simulink model "AR_Drone_Flight_Control"  (R2014a)
settings: configuration reference "AR_Drone_ConfigSet" (kept outside this file)
values from neighbouring files (symbols this model uses):
  Accelerometer_quick_calibration = [0.003485 0.008674 -0.9985]    [Calibration_Parameters.mat]
  Gyrometer_quick_calibration = [-10.63 2.778 -0.1868]    [Calibration_Parameters.mat]
undefined symbols (not defined in the file or in its folder): Accelerometer_360deg_calibration, Drone_StateModeType, Magnetometer_calibration, Navigation, Navigation_KF_Lib, sigbuilder_block
libraries: simulink x15, vrlib x7, aerolibtransform2 x5, AR_Drone_2_Library x4, dspnetwork x3, aerolibutil x2
(part 2 of 3)

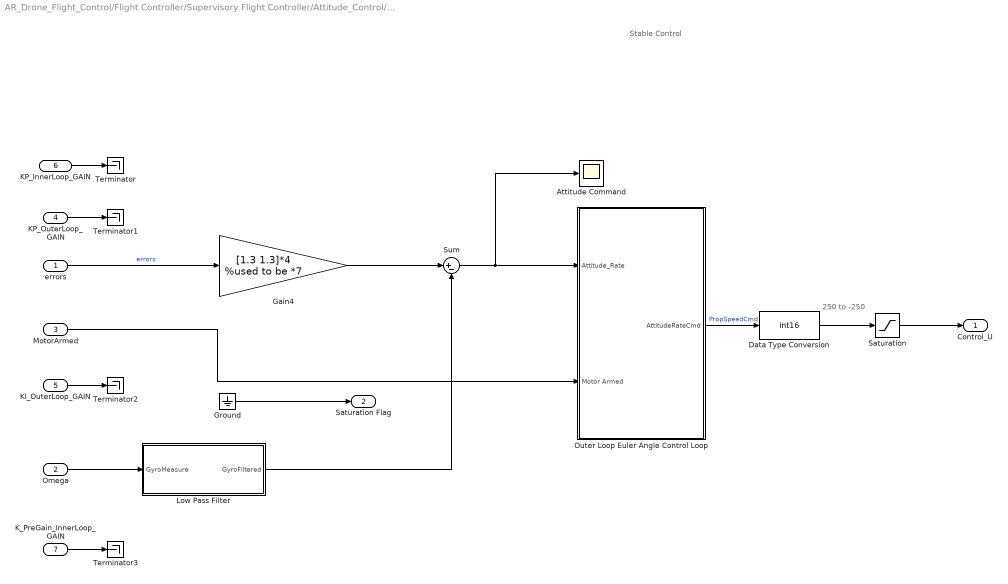
== system AR_Drone_Flight_Control/Flight Controller/Supervisory Flight Controller/Attitude_Control/Roll Pitch Controller ==
  note: 250 to -250
  note: Stable Control
  errors : Inport
  Omega : Inport  Port=2
  MotorArmed : Inport  Port=3
  KP_OuterLoop_GAIN : Inport  Port=4
  KI_OuterLoop_GAIN : Inport  Port=5
  KP_InnerLoop_GAIN : Inport  Port=6
  K_PreGain_InnerLoop_GAIN : Inport  Port=7
  Attitude Command : Scope
      settings: SaveName=AttitudeRateCtrl_Cmd
  Data Type Conversion : DataTypeConversion  OutDataTypeStr=int16  RndMeth=Nearest
  Gain4 : Gain  Gain="[1.3 1.3]*4  %used to be *7"
  Ground : Ground
  Low Pass Filter : Subsystem
  Outer Loop Euler Angle Control Loop : Subsystem
  Saturation : Saturate  UpperLimit=250  LowerLimit=-250  OutDataTypeStr=int16
      settings: AttributesFormatString=%<LowerLimit>\nto\n%<UpperLimit>
  Sum : Sum  Inputs=|+-
  Terminator{,1..3} (4 alike) : Terminator
  Control_U : Outport
  Saturation Flag : Outport  Port=2
  wires:
  Saturation/1 -> Control_U/1
  Data Type Conversion/1 -> Saturation/1
  Outer Loop Euler Angle Control Loop/1(AttitudeRateCmd) -> Data Type Conversion/1  "PropSpeedCmd"
  MotorArmed/1 -> Outer Loop Euler Angle Control Loop/2(Motor Armed)
  Ground/1 -> Saturation Flag/1
  Omega/1 -> Low Pass Filter/1(GyroMeasure)
  errors/1 -> Gain4/1  "errors"
  Sum/1 -> Attitude Command/1, Outer Loop Euler Angle Control Loop/1(Attitude_Rate)
  Gain4/1 -> Sum/1
  Low Pass Filter/1(GyroFiltered) -> Sum/2
  KP_InnerLoop_GAIN/1 -> Terminator/1
  KP_OuterLoop_GAIN/1 -> Terminator1/1
  KI_OuterLoop_GAIN/1 -> Terminator2/1
  K_PreGain_InnerLoop_GAIN/1 -> Terminator3/1

== system AR_Drone_Flight_Control/Flight Controller/Supervisory Flight Controller/Attitude_Control/Yaw Counter-Active Control ==
  note: This Yaw Controller will prevent the drone from
      | rotating but does not tell the drone to rotate to a specified angle
  Euler_Yaw_Deg : Inport
  Rate_Gyro_R_deg : Inport  Port=2
  "Desired_yaw " : Inport  Port=3
  Add1 : Sum  Inputs=+-  AccumDataTypeStr=single  OutDataTypeStr=single
  Add2 : Sum  Inputs=+-  AccumDataTypeStr=single  OutDataTypeStr=single
  Data Type Conversion : DataTypeConversion  OutDataTypeStr=int16
  Discrete Derivative : simulink/Discrete/Discrete Derivative  gainval=1.0  ICPrevScaledInput=0.0  InputProcessing=Inherited  OutMin=[]  OutMax=[]  OutDataType=fixdt(1, 16)  OutScaling=2^-10  DoSatur=off
  InterChange_Axis : Gain  Gain=-1  ParamDataTypeStr=single  OutDataTypeStr=single
      settings: AttributesFormatString=%<Gain>
  To Degrees2 : Gain  Gain=180/pi  ParamDataTypeStr=single  OutDataTypeStr=single
      settings: AttributesFormatString=%<Gain>
  To Degrees3 : Gain  ParamDataTypeStr=single  OutDataTypeStr=single
      settings: AttributesFormatString=%<Gain>
  Yaw_contribution : Gain  Gain=2.5*2  ParamDataTypeStr=single  OutDataTypeStr=single
      settings: AttributesFormatString=%<Gain>
  Yaw_contribution1 : Gain  Gain=0.06  ParamDataTypeStr=single  OutDataTypeStr=single
      settings: AttributesFormatString=%<Gain>
  YawCommand : Outport
  wires:
  Yaw_contribution1/1 -> Data Type Conversion/1
  To Degrees3/1 -> Add1/2
  Euler_Yaw_Deg/1 -> InterChange_Axis/1
  Add1/1 -> Yaw_contribution1/1
  Yaw_contribution/1 -> Add1/1
  Add2/1 -> Yaw_contribution/1
  InterChange_Axis/1 -> Discrete Derivative/1
  Discrete Derivative/1 -> Add2/1
  To Degrees2/1 -> Add2/2
  "Desired_yaw "/1 -> To Degrees2/1
  Rate_Gyro_R_deg/1 -> To Degrees3/1
  Data Type Conversion/1 -> YawCommand/1

== system AR_Drone_Flight_Control/Flight Controller/Supervisory Flight Controller/Attitude_Control/Yaw Signal Builder  ==
  Demux : Demux  Tag=STV Demux  Outputs=1
  FromWs : FromWorkspace  Tag=STV FromWs  VariableName=tuvar
      SigBuilderData=|
      | common.afterFinalStr = 'Extrapolate'
      | common.sampleTime = '-1'
      | dataSet.timeRange = [0 20]
      | dataSet.name = 'Group 1'
      | sbobj.Groups.Name = 'Group 1'
      | sbobj.Groups.Signals.Name = 'Signal 1'
      | sbobj.Groups.Signals.XData = [0 10 10 12.5 12.5 15 15 20]
      | sbobj.Groups.Signals.YData = [0 0 2 2 -2 -2 0 0]
      | sbobj.Groups.TimeRange = [0 20]
  Signal 1 : Outport  Tag=STV Outport
  wires:
  Demux/1 -> Signal 1/1
  FromWs/1 -> Demux/1

== stateflow chart AR_Drone_Flight_Control/Navigation/CheckSum Pre-Processing/Ultrasound Processing/CheckSum Correction/Generate Sample Holding Pulse/Chart ==
  state Begin_State0
    entry: output =0;
  state Begin_State
    entry: output =1;
  state End_State
    entry: output=0;
  (default) -> Begin_State0
  Begin_State0 -> Begin_State : [if_transition==1]
  Begin_State -> End_State [order 1] : after(HoldDataTicks,tick)
  End_State -> Begin_State : [if_transition==1]
  Begin_State -> Begin_State [order 2] : [if_transition==1]
  data: output output; if_transition input; HoldDataTicks input

== matlab function AR_Drone_Flight_Control/Navigation/CheckSum Pre-Processing/Ultrasound Processing/Height Calculation ==
  data: u input double; y output double; prev_good_height output double; z_1 input double
function [y,prev_good_height] = fcn(u,z_1)
%#codegen



if u<10000
    
    height = ((u - 880) /26.553);
    prev_good_height = height;
else
    
%     height = u;
%     prev_good_height = height;
    height =  z_1;
    prev_good_height = z_1; 
end

y = height;

== stateflow chart AR_Drone_Flight_Control/Flight Controller/Supervisory Flight Controller ==
  state Fault_Check [parallel]
    settings: executionOrder=3
    state BatteryFault_Check [parallel]
      settings: executionOrder=1
      state BatteryNominal
        en:
        BatteryFault = 0;
        state Nominal
        note: Description:
            | This state will be responsible for the following
            |
            | - Automatically land the drone by forcing it to the land state when voltage is low
            | - Prevent drone from taking off if battery voltage is too low
        state EvaluateVoltageLevel
        state ChangeState
          en:
          BatteryFault = 1;
        EvaluateVoltageLevel -> Fault_Check.BatteryFault_Check.BatteryNominal.Nominal [order 1] : [Measured_Battery_Voltage>=10.1]
        Fault_Check.BatteryFault_Check.BatteryNominal.Nominal -> EvaluateVoltageLevel : [Measured_Battery_Voltage<10.1]
        (default) -> EvaluateVoltageLevel
        EvaluateVoltageLevel -> Fault_Check.BatteryFault_Check.BatteryNominal.ChangeState [order 2] : after(5,sec)
      state BatteryLow
        state ForceLanding
          en:
        (default) -> ForceLanding
      (default) -> BatteryNominal
      BatteryNominal -> BatteryLow : [BatteryFault==1]
    state UltraSoundwarning_Check [parallel]
      settings: executionOrder=2
    state SafeOrientation_Check [parallel]
      settings: executionOrder=3
      state UnsafeOrientation
        du:
        MotorArmed =0;
        LandingPhase = 0;
      state WaitForFlight
      state GravityVectorCheck
        en:
        OrientationFault = 0;
        note: Description:
            | This state will be responsible for the following
            |
            | - Automatically land the drone by forcing it to the land state when voltage is low
            | - Prevent drone from taking off if battery voltage is too low
        state Nominal
        state EvaluateGravityVector
        state ChangeState
          en:
          OrientationFault = 1;
        EvaluateGravityVector -> Fault_Check.SafeOrientation_Check.GravityVectorCheck.Nominal [order 1] : [AccelVector_Input<-0.05]
        Fault_Check.SafeOrientation_Check.GravityVectorCheck.Nominal -> EvaluateGravityVector : [AccelVector_Input>=0.05]
        (default) -> EvaluateGravityVector
        EvaluateGravityVector -> Fault_Check.SafeOrientation_Check.GravityVectorCheck.ChangeState [order 2] : after(0.01,sec)
      (default) -> WaitForFlight
      GravityVectorCheck -> WaitForFlight [order 2] : [in(Drone_State.WaitForHost)]
      GravityVectorCheck -> UnsafeOrientation [order 1] : [OrientationFault ==1]
      WaitForFlight -> GravityVectorCheck : [in(Drone_State.Controlled_Flight)]
  state Drone_State [parallel]
    settings: executionOrder=1
    state WaitForHost
      entry:
      reset_offset_calc = 0;
      MotorArmed = 0;
      refHeight = 0;
      LandingPhase = 0;
      Flight_Mission_On_Off = false;
      note: Description:
          | -This state will wait for the host command to take off, while initializing the offsets (accel & gyro)
          |
          | -Upon entry, this block will set the motor to NOT ARMED (turn off integrators in controller, set safety clamp of motors to OFF)
          | -Upon entry, set the refHeight to ZERO
          | -Upon entry, reset the offset calculation such that we can re-start the averaging block
      state converge = checkConvergence(Euler_Angles) [function]
      state move = checkMove(Euler_Angles) [function]
      state Attitude_Convergence_Wait
        entry:
        initDone=false;
        during:
        Converge_Flag = checkConvergence(Gyro_Measures_for_Offset);
      state Calculate_Attitude_Offset
        entry:
        reset_offset_calc = 0 ;
        Move = false;
        during:
        Offset_Accel_Current =Accel_Offset_Calculation(Accel_Measures_for_Offset,reset_offset_calc);
        Offset_Gyro_Current =Gyro_Offset_Calculation(Gyro_Measures_for_Offset,reset_offset_calc);
        Move = checkMove(Gyro_Measures_for_Offset);
      state Wait_For_Flight
        entry:
        Offset_Accel = Accelerometer_quick_calibration;
        Offset_Gyro = Gyrometer_quick_calibration;
        during:
        initDone = true;
      state Auto_Calibration_Done
        entry:
        Offset_Accel = Offset_Accel_Current;
        Offset_Gyro = Offset_Gyro_Current;
        reset_offset_calc = 1;
        Accel_Offset_Calculation(Accel_Measures_for_Offset,reset_offset_calc);
        Gyro_Offset_Calculation(Gyro_Measures_for_Offset,reset_offset_calc);
        during:
        initDone = true;
      (default) -> Attitude_Convergence_Wait
      Calculate_Attitude_Offset -> Attitude_Convergence_Wait [order 2] : [Move == 1 && after(0.1,sec)]
          | {reset_offset_calc = 1;
          | Accel_Offset_Calculation(Accel_Measures_for_Offset,reset_offset_calc);
          | Gyro_Offset_Calculation(Gyro_Measures_for_Offset,reset_offset_calc)}
      Auto_Calibration_Done -> Attitude_Convergence_Wait [order 2] : [Auto_Calibration==false]
      Wait_For_Flight -> Attitude_Convergence_Wait : [Auto_Calibration==true]
      Attitude_Convergence_Wait -> (junction 628) : [Converge_Flag==1 && after(0.1,sec)]
      (junction 628) -> Calculate_Attitude_Offset [order 1] : [Auto_Calibration==true]
      (junction 628) -> Wait_For_Flight [order 2] : [Auto_Calibration==false]
      Calculate_Attitude_Offset -> Auto_Calibration_Done [order 1] : [Move == 0 && after(3,sec)]
      Auto_Calibration_Done -> Calculate_Attitude_Offset [order 1] : [initDone == 1 && after(0.1,sec)]
    state Controlled_Flight
      entry:
      LandingPhase = 0;
      MotorArmed =1;
      note: Description:
          | -Upon entry, this block will set the motor to ARMED (enable controller integrator and motor safetey unclamped)
          | -This block will command the AR Drone to fly up to a certain height using the variable refHeight
          | -The output of refHeight should be a function of desired Altitude. The most primitive assignment is to make refHeight = DesiredAltitude, this is comparable to giving the drone a step response. Alternate methods could be giving it a smooth trajectory to follow from the ground to that particular height
          |
          | -Below is an example of what it might look like
      state Initialize
        entry: refHeight = 0;
      state Altitude_Climb
        entry: Flight_Mission_On_Off = true;
        during: Input_ports = [0 ; 0];
        refHeight = Output_ports(2);
      (default) -> Initialize
      Initialize -> Altitude_Climb : [after(0.5,sec)]
    state Landing_Sequence
      entry:
      refHeight = min(refHeight,40);
      Flight_Mission_On_Off = false;
      note: Description:
          | -Entry into this state will occur if
          | a) Battery drops to around 10.5-10.2 Volts (needs to be experimentally validated)
          | b) Entry condition is met from the user input
          | c) Attitude is out of bounds, ie: the quad rotor has tilted it's pitch to some uncontrollable angle such as 80 degrees
          |
          | Substate goals:
          | -Descend at a controllable rate and land safely
      state Climb_down_1
        entry: refHeight = refHeight - 2 ;
      state Climb_down_2
        entry: refHeight = refHeight - 1 ;
      state Climb_down_3
        entry: LandingPhase=1;
      (default) -> Climb_down_1
      Climb_down_1 -> Climb_down_1 [order 1] : [UltraSound_Feedback(1) <= refHeight && after(0.05,sec)]
      Climb_down_1 -> Climb_down_2 [order 2] : [UltraSound_Feedback(1) <= 10 && after(0.1,sec)]
      Climb_down_2 -> Climb_down_2 [order 1] : [UltraSound_Feedback(1) <= refHeight && after(0.1,sec)]
      Climb_down_2 -> Climb_down_3 [order 2] : [UltraSound_Feedback(1) <= 0.5 && after(0.1,sec)]
    state Landing_Terminate
      entry:
      MotorArmed =0;
      LandingPhase = 0;
      Flight_Mission_On_Off = false;
      %Catch any last state action we need to do here
      note: Description:
          | This state is optional and might not be needed. Up to you if you think having an extra state for the landing phase might be useful.. if not, delete it and consolidate it into previous state
    (default) -> WaitForHost
    Landing_Terminate -> WaitForHost : [sum(MotorCmd)==0]
    WaitForHost -> Controlled_Flight : [ (hostCmd == Drone_StateModeType.Controlled_Flight)...
        |  &&...
        |  in(Fault_Check.BatteryFault_Check.BatteryNominal.Nominal)...
        | && (initDone == 1) ]
    Controlled_Flight -> Landing_Terminate [order 2] : [in(Fault_Check.SafeOrientation_Check.UnsafeOrientation)]
    Controlled_Flight -> Landing_Sequence [order 1] : [(hostCmd == ...
        | Drone_StateModeType.Landing_Sequence)...
        | ||...
        |  in(Fault_Check.BatteryFault_Check.BatteryLow) ]
    Landing_Sequence -> Landing_Terminate : [sum(MotorCmd)==0]
  state Flight_Controls [parallel]
    settings: executionOrder=2
    state Attitude_Command [parallel]
      entry, during:
      Attitude_Thrust = Attitude_Control(Desired_Attitude_deg,Euler_Angles,Angular_Velocity,MotorArmed);
      settings: executionOrder=1
    state Altitude_Command [parallel]
      entry, during:
      Altitude_Thrust = Altitude_Control(UltraSound_Feedback,refHeight);
      settings: executionOrder=2
    state MotorMixing_Command [parallel]
      entry, during:
      throttle = NominalThrust+EnableAltitudeCtrl*Altitude_Thrust;
      MotorCmd = Motor_Mixing(throttle,Attitude_Thrust,LandingPhase,MotorArmed);
      settings: executionOrder=3
  state deltaThrottle = Altitude_Control(HeightFeedback,refHeight) [function]
  state controls = Attitude_Control(Desired_Attitude_Deg,EulerAngle_Feedback_Deg,RateGyro_Feedback_Deg,Motor_Armed) [function]
  state MotorCommands = Motor_Mixing(throttle,RPYCmd,LandingPhase,Motor_Armed) [function]
  data: Euler_Angles function_input double size=3; converge function_output; OffsetMeasure function_input; Reset function_input; Y function_output; OffsetMeasure function_input; Reset function_input; Y function_output; Euler_Angles function_input double size=3; move function_output; HeightFeedback function_input double size=2; refHeight function_input double size=1; deltaThrottle function_output int16; Desired_Attitude_Deg function_input double size=3; EulerAngle_Feedback_Deg function_input double size=3; RateGyro_Feedback_Deg function_input double size=3; Motor_Armed function_input double size=1; controls function_output int16 size=3; throttle function_input int16 size=1; RPYCmd function_input int16 size=3; LandingPhase function_input double size=1; MotorCommands function_output; Motor_Armed function_input double size=1; hostCmd input Enum: Drone_StateModeType; Auto_Calibration input; EnableAltitudeCtrl input; Desired_Attitude_deg input size=3; UltraSound_Feedback input size=2; initDone local; MotorCmd output size=4; throttle local int16; deltaThrottle local; height local; Euler_Angles input; Angular_Velocity input; AccelVector_Input input; hoverHeight local; NominalThrust input; Drone_StateMode output Enum: Drone_StateModeType; Measured_Battery_Voltage input; Attitude_Thrust local; Altitude_Thrust local; Converge_Flag local; reset_offset_calc local; MotorArmed local; Offset_Accel data_store_memory; LandingPhase local; N local; Accel_Measures_for_Offset input size=3; Gyro_Measures_for_Offset input size=3; Offset_Gyro data_store_memory; Offset_Gyro_Current local; Offset_Value_Current local; Offset_Accel_Current local double; BatteryFault local; OrientationFault local; BatteryFault_Mode output Enum: BatteryFault_ModeType; SafeOrientation_Mode output Enum: SafeOrientation_ModeType; refHeight output; Move local; Landing_Altitude local; Actual_Attitude local; Gyrometer_quick_calibration parameter; Accelerometer_quick_calibration parameter; Flight_Mission_On_Off data_store_memory; Output_ports data_store_memory; Input_ports data_store_memory
  data hostCmd settings: description=|
      | The hostCmd can take the values 0,1 and 2.
      | 
      | 0 - default state when the drone is powered up.
      | 1 - Takeoff
      | 2 - Landing
  data EnableAltitudeCtrl settings: description=A flag to enable the altitude controller
  data UltraSound_Feedback settings: description=Ultrasound Feedback will contain data on current height (cm) and altitude rate (cm/s)
  data initDone settings: description=A flag to check whether the calibration is done.
  data NominalThrust settings: description=Nominal thrust input (approximately 60% duty cycle)
  data refHeight settings: description=Desired height at which the drone needs to hover.
  function Y = Accel_Offset_Calculation(OffsetMeasure,Reset):
    | function Y = Accel_Offset_Calculation(OffsetMeasure,Reset)
    |  
    | %Compute running average while in this state. Assumed inputs
    | %are accelerometer offset values. These values are accumulated over time
    | %and divided by the total time increment to return an average values
    | Y = [0 0 0]';
    | persistent A_x_sum
    | persistent A_y_sum
    | persistent A_z_sum
    | persistent Tick
    | 
    | if(isempty(A_x_sum) || Reset==1)
    |     A_x_sum = 0;
    |     A_y_sum = 0;
    |     A_z_sum = 0;
    |     Tick = 1;
    |         
    | else
    |     
    |     Measure_X = OffsetMeasure(1);
    |     Measure_Y = OffsetMeasure(2);
    |     Measure_Z = OffsetMeasure(3);
    | 
    |     A_x_sum = A_x_sum + Measure_X;
    |     A_y_sum = A_y_sum + Measure_Y;
    |     A_z_sum = A_z_sum + Measure_Z;
    | 
    | 
    |     Y = [A_x_sum A_y_sum A_z_sum]'./Tick;
    | 
    | 
    |     Tick = Tick + 1;
    | 
    | end
    | 
    | 
    | 
    | 
    | end
  function Y = Gyro_Offset_Calculation(OffsetMeasure,Reset):
    | function Y = Gyro_Offset_Calculation(OffsetMeasure,Reset)
    |  
    | %Compute running average while in this state. Assumed inputs
    | %are gyro offset values when drone is perfectly stationary on the ground. These values are accumulated over time
    | %and divided by the total time increment to return an average values
    | Y = [0 0 0]';
    | persistent G_x_sum
    | persistent G_y_sum
    | persistent G_z_sum
    | persistent Tick
    | 
    | if(isempty(G_x_sum) || Reset==1)
    |     G_x_sum = 0;
    |     G_y_sum = 0;
    |     G_z_sum = 0;
    | 
    |     Tick = 1;
    |         
    | else
    |     
    |     Measure_X = OffsetMeasure(1);
    |     Measure_Y = OffsetMeasure(2);
    |     Measure_Z = OffsetMeasure(3);
    | 
    |     G_x_sum = G_x_sum + Measure_X;
    |     G_y_sum = G_y_sum + Measure_Y;
    |     G_z_sum = G_z_sum + Measure_Z;
    | 
    | 
    |     Y = [G_x_sum G_y_sum G_z_sum]'./Tick;
    | 
    | 
    |     Tick = Tick + 1;
    | 
    | end
    | 
    | 
    | 
    | 
    | end

== system AR_Drone_Flight_Control/Flight Mission/Desired Drone_StateMode Management/Data Correction ==
  note: This Subsystem tests if the data is normal (it should be equal to -1 or +1)
      | If not (for exemple if the UDP server waits data but receives nothing : 0),
      | it affects to the data the last "normal" value seen (initial condition : -1)
  Start/Stop : Inport
  Constant1 : Constant  Value=-1
  Constant2 : Constant  Value=+1
  Logical Operator : Logic  Operator=OR  AllPortsSameDT=off  OutDataTypeStr=boolean
  Memory : Memory  X0=-1
  Switch1 : Switch  Criteria=u2 > Threshold
  Tests if data equals +1 : RelationalOperator  Operator===  OutDataTypeStr=boolean
  Tests if data equals -1 : RelationalOperator  Operator===  OutDataTypeStr=boolean
  Real Start/Stop : Outport
  wires:
  Start/Stop/1 -> Switch1/1, Tests if data equals -1/2, Tests if data equals +1/1
  Constant1/1 -> Tests if data equals -1/1
  Constant2/1 -> Tests if data equals +1/2
  Tests if data equals -1/1 -> Logical Operator/1
  Tests if data equals +1/1 -> Logical Operator/2
  Logical Operator/1 -> Switch1/2
  Switch1/1 -> Memory/1, Real Start/Stop/1
  Memory/1 -> Switch1/3

== system AR_Drone_Flight_Control/Navigation/CheckSum Pre-Processing/Accelerometer Processing ==
  Raw Data : Inport
  CheckSum Flag : Inport  Port=2
  Holding Value : Inport  Port=3
  Calculate Accel Data : Subsystem  Commented=through
  CheckSum Correction : Subsystem
  Processed Data : Outport
  wires:
  Holding Value/1 -> CheckSum Correction/3(Holding Value)
  Calculate Accel Data/1(Processed Accel Data) -> CheckSum Correction/1(CalculatedData)
  CheckSum Correction/1(Pre-Processed Height) -> Processed Data/1
  Raw Data/1 -> Calculate Accel Data/1(Raw Accel Data)
  CheckSum Flag/1 -> CheckSum Correction/2(CheckSumFlag)

== system AR_Drone_Flight_Control/Navigation/CheckSum Pre-Processing/Magnetometer ==
  Magnetometer : Inport
  CheckSum Flag : Inport  Port=2
  Holding Value : Inport  Port=3
  CheckSum Correction : Subsystem
  Process Raw Mag Data : Subsystem  Commented=through
  Processed Data : Outport
  wires:
  Holding Value/1 -> CheckSum Correction/3(Holding Value)
  Process Raw Mag Data/1(ProcessedData) -> CheckSum Correction/1(CalculatedData)
  Magnetometer/1 -> Process Raw Mag Data/1(Magnetometer)
  CheckSum Correction/1(Pre-Processed Data) -> Processed Data/1
  CheckSum Flag/1 -> CheckSum Correction/2(CheckSumFlag)

== system AR_Drone_Flight_Control/Navigation/CheckSum Pre-Processing/RateGyro Processing ==
  Raw Data : Inport
  CheckSum Flag : Inport  Port=2
  Holding Value : Inport  Port=3
  CheckSum Correction : Subsystem
  Process Data : Subsystem  Commented=through
  Processed Data : Outport
  wires:
  Holding Value/1 -> CheckSum Correction/3(Holding Value)
  Process Data/1(Processed Data) -> CheckSum Correction/1(CalculatedData)
  Raw Data/1 -> Process Data/1(Raw Data)
  CheckSum Correction/1(Pre-Processed Height) -> Processed Data/1
  CheckSum Flag/1 -> CheckSum Correction/2(CheckSumFlag)

== system AR_Drone_Flight_Control/Navigation/CheckSum Pre-Processing/TempFilter ==
  Magnetometer : Inport
  CheckSum Flag : Inport  Port=2
  HoldingValue : Inport  Port=3
  CheckSum Correction : Subsystem
  Process Raw Mag Data : Subsystem  Commented=through
  Processed Data : Outport
  wires:
  HoldingValue/1 -> CheckSum Correction/3(Holding Value)
  Process Raw Mag Data/1(ProcessedData) -> CheckSum Correction/1(CalculatedData)
  Magnetometer/1 -> Process Raw Mag Data/1(Magnetometer)
  CheckSum Correction/1(Pre-Processed Data) -> Processed Data/1
  CheckSum Flag/1 -> CheckSum Correction/2(CheckSumFlag)

== system AR_Drone_Flight_Control/Navigation/CheckSum Pre-Processing/Ultrasound Processing ==
  note: '192.168.1.1' 1 17725
  Raw Ultrasound : Inport
  CheckSum Flag : Inport  Port=2
  Holding Value : Inport  Port=3
  CheckSum Correction : Subsystem
  Data Type Conversion1 : DataTypeConversion
  Delay1 : Delay  DelayLength=1  InitialCondition=0
  Height Calculation : MATLAB Function  TreatAsAtomicUnit=on
  Saturation1 : Saturate  UpperLimit=100e3  LowerLimit=0
  Processed Data : Outport
  wires:
  Holding Value/1 -> CheckSum Correction/3(Holding Value)
  Saturation1/1 -> Processed Data/1
  CheckSum Correction/1(Pre-Processed Height) -> Saturation1/1
  CheckSum Flag/1 -> CheckSum Correction/2(CheckSumFlag)
  Height Calculation/1(y) -> CheckSum Correction/1(CalculatedData)
  Raw Ultrasound/1 -> Data Type Conversion1/1
  Height Calculation/2(prev_good_height) -> Delay1/1
  Data Type Conversion1/1 -> Height Calculation/1(u)
  Delay1/1 -> Height Calculation/2(z_1)

== system AR_Drone_Flight_Control/Navigation/Data Conversion and Measurement Calculation/Calculate Gravity Vector ==
  Accel : Inport
  Accel_Offset : Inport  Port=2
  Accelerometer Neutral Gain and Offset : Subsystem
  Calibration_GainOffset : Subsystem
  Compare Calibration : Scope  NumInputPorts=2
      settings: TimeRange=6.848856838354834  YMin=-1.05~-1.05  YMax=0.05~0.1  SaveName=AccelProcessed_Record1
  Compare Filter : Scope  NumInputPorts=2
      settings: TimeRange=6.848856838354834  YMin=-0.05~-0.05  YMax=1.05~1.05  SaveName=AccelProcessed_Record2
  Compare Offset : Scope  NumInputPorts=2
      settings: TimeRange=6.848856838354834  YMin=-0.05~-1  YMax=1.05~0.05  SaveName=AccelProcessed_Record
  InitialCondition_Offset : Subsystem
  Low Pass Filter : Subsystem
  Normalize Vector : vrlib/Utilities/Normalize Vector  maxzero=0
  Accel_Norm : Outport
  wires:
  Accel_Offset/1 -> InitialCondition_Offset/2(Accel_Offset)
  Accelerometer Neutral Gain and Offset/1(Processed Accel Data) -> Compare Calibration/2, Calibration_GainOffset/1(Pre)
  Calibration_GainOffset/1(Post) -> Compare Offset/2, Compare Calibration/1, InitialCondition_Offset/1(Pre)
  Low Pass Filter/1(Filtered Accel) -> Normalize Vector/1, Compare Filter/1
  InitialCondition_Offset/1(Post) -> Low Pass Filter/1(Offset Accel), Compare Filter/2, Compare Offset/1
  Accel/1 -> Accelerometer Neutral Gain and Offset/1(Raw Accel Data)
  Normalize Vector/1 -> Accel_Norm/1

== system AR_Drone_Flight_Control/Navigation/Data Conversion and Measurement Calculation/Calibration_Scale_and_Offset ==
  RawMag : Inport
  Normalize Vector : vrlib/Utilities/Normalize Vector  maxzero=0
  Process Raw Mag Data : Subsystem  Variant=on  OverrideUsingVariant=TempVariantA
  Normalized  Magnetometer : Outport
  wires:
  Process Raw Mag Data/1(MagVector) -> Normalize Vector/1
  RawMag/1 -> Process Raw Mag Data/1(Magnetometer)
  Normalize Vector/1 -> Normalized  Magnetometer/1

== system AR_Drone_Flight_Control/Navigation/Data Conversion and Measurement Calculation/Remove Offset ==
  Raw Gyro Values : Inport
  Gyro Offset : Inport  Port=2
  BeforeAfter : Scope
      settings: YMin=-40  YMax=40
  Demux : Demux  Outputs=3
  Demux1 : Demux  Outputs=3
  Display : Display
  Mux : Mux  Inputs=2
  Mux1 : Mux  Inputs=3
  Process Raw Rate Gyro Data : Subsystem
  Sum : Sum  Inputs=|+-
  Sum1 : Sum  Inputs=|+-
  Sum2 : Sum  Inputs=|+-
  Gyro Offset Remove : Outport
  tag scope: Gyro_data_for_offset=global
  wires:
  Process Raw Rate Gyro Data/1(Processed Data) -> Gyro Offset Remove/1
  Mux/1 -> BeforeAfter/1
  Raw Gyro Values/1 -> Demux/1, Mux/1, [Gyro_data_for_offset]
  Gyro Offset/1 -> Demux1/1
  Mux1/1 -> Process Raw Rate Gyro Data/1(Raw Rate Gyro Data), Display/1, Mux/2
  Demux1/3 -> Sum2/2
  Demux1/2 -> Sum1/2
  Demux1/1 -> Sum/2
  Demux/2 -> Sum1/1
  Demux/1 -> Sum/1
  Sum1/1 -> Mux1/2
  Demux/3 -> Sum2/1
  Sum2/1 -> Mux1/3
  Sum/1 -> Mux1/1

== system AR_Drone_Flight_Control/Navigation/SL3D Visualization/Interchange Axes Accel for SL3D  ==
  VRML_in : Inport
  Demux1 : Demux  Outputs=3
  Gain1 : Gain  Gain=3
  Gain2 : Gain
  Gain3 : Gain
  Mux2 : Mux  Inputs=3
  VRML_out : Outport
  wires:
  VRML_in/1 -> Gain1/1
  Demux1/2 -> Gain2/1
  Mux2/1 -> VRML_out/1
  Gain3/1 -> Mux2/3
  Gain2/1 -> Mux2/1
  Demux1/3 -> Mux2/2
  Demux1/1 -> Gain3/1
  Gain1/1 -> Demux1/1

== system AR_Drone_Flight_Control/Navigation/SL3D Visualization/Interchange Axes Mag for SL3D  ==
  VRML_in : Inport
  Home Drone : Subsystem
  Subsystem : Subsystem  Commented=on
  Work Drone : Subsystem
  Work Drone - supposed work drone .. not really : Subsystem
  VRML_out : Outport
  wires:
  Work Drone/1(Out1) -> VRML_out/1
  VRML_in/1 -> Home Drone/1(In1), Work Drone/1(In1)

== system AR_Drone_Flight_Control/Navigation/SL3D Visualization/Interchange Axis Mag Project for SL3D ==
  VRML_in : Inport
  Demux1 : Demux  Outputs=3
  Gain2 : Gain
  Gain3 : Gain
  Mux2 : Mux  Inputs=3
  VRML_out : Outport
  wires:
  Demux1/2 -> Gain2/1
  Mux2/1 -> VRML_out/1
  Gain3/1 -> Mux2/3
  Gain2/1 -> Mux2/1
  Demux1/3 -> Mux2/2
  Demux1/1 -> Gain3/1
  VRML_in/1 -> Demux1/1

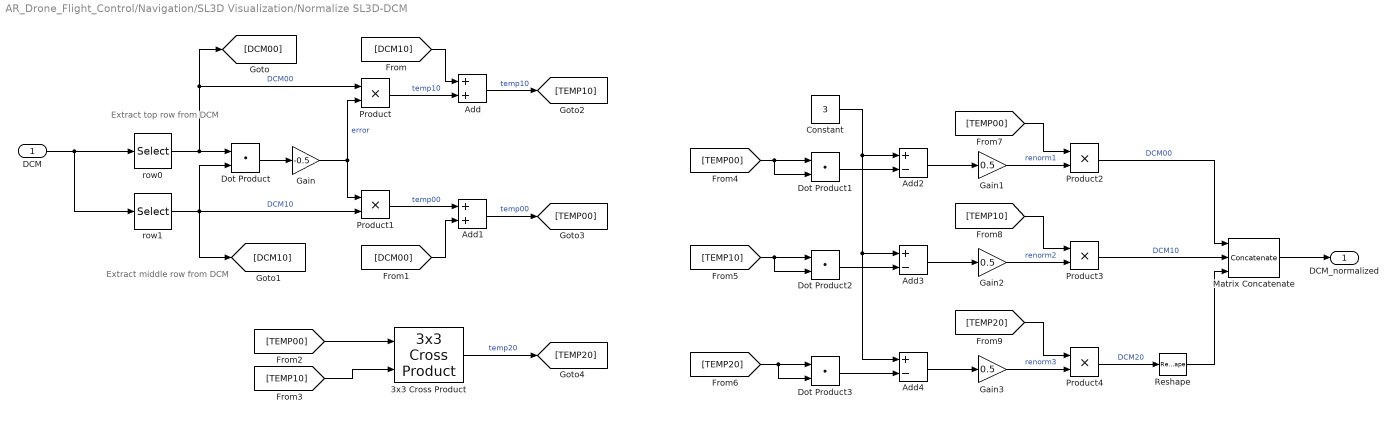
== system AR_Drone_Flight_Control/Navigation/SL3D Visualization/Normalize SL3D-DCM ==
  note: Extract top row from DCM
  note: Extract middle row from DCM
  DCM : Inport  OutDataTypeStr=double  PortDimensions=[3,3]
  3x3 Cross Product : aerolibutil/3x3 Cross Product
  Add : Sum
  Add1 : Sum
  Add2 : Sum  Inputs=+-
  Add3 : Sum  Inputs=+-
  Add4 : Sum  Inputs=+-
  Constant : Constant  Value=3  OutDataTypeStr=double  SampleTime=-1
  Dot Product{,1..3} (4 alike) : DotProduct  InputSameDT=on  OutDataTypeStr=Inherit: Inherit via internal rule
  Gain : Gain  Gain=-0.5
  Gain1 : Gain  Gain=0.5  OutDataTypeStr=single
  Gain2 : Gain  Gain=0.5  OutDataTypeStr=single
  Gain3 : Gain  Gain=0.5  OutDataTypeStr=single
  Matrix Concatenate : Concatenate  NumInputs=3  Mode=Multidimensional array
  Product{,1..4} (5 alike) : Product  RndMeth=Zero
  Reshape : Reshape  OutputDimensionality=Row vector (2-D)
  row0 : Selector  NumberOfDimensions=2  IndexMode=Zero-based  InputPortWidth=3  IndexOptions=Index vector (dialog),Index vector (dialog)  Indices=0,[0:2]  OutputSizes=1,1
  row1 : Selector  NumberOfDimensions=2  IndexMode=Zero-based  InputPortWidth=3  IndexOptions=Index vector (dialog),Index vector (dialog)  Indices=1,[0:2]  OutputSizes=1,1
  DCM_normalized : Outport  OutDataTypeStr=double
  wires:
  DCM/1 -> row0/1, row1/1
  row0/1 -> Dot Product/1, Product/1, [DCM00]  "DCM00"
  row1/1 -> Dot Product/2, Product1/2, [DCM10]  "DCM10"
  Dot Product/1 -> Gain/1
  Gain/1 -> Product/2, Product1/1  "error"
  Product/1 -> Add/2  "temp10"
  Product1/1 -> Add1/1  "temp00"
  [DCM10] -> Add/1
  [DCM00] -> Add1/2
  Add/1 -> [TEMP10]  "temp10"
  Add1/1 -> [TEMP00]  "temp00"
  3x3 Cross Product/1 -> [TEMP20]  "temp20"
  [TEMP00] -> 3x3 Cross Product/1
  [TEMP10] -> 3x3 Cross Product/2
  [TEMP00] -> Dot Product1/1, Dot Product1/2
  [TEMP10] -> Dot Product2/1, Dot Product2/2
  [TEMP20] -> Dot Product3/1, Dot Product3/2
  Dot Product1/1 -> Add2/2
  Constant/1 -> Add2/1, Add4/1, Add3/1
  Add2/1 -> Gain1/1
  Gain1/1 -> Product2/2  "renorm1"
  Add3/1 -> Gain2/1
  Gain2/1 -> Product3/2  "renorm2"
  Dot Product2/1 -> Add3/2
  Add4/1 -> Gain3/1
  Gain3/1 -> Product4/2  "renorm3"
  Dot Product3/1 -> Add4/2
  [TEMP00] -> Product2/1
  [TEMP10] -> Product3/1
  [TEMP20] -> Product4/1
  Product2/1 -> Matrix Concatenate/1  "DCM00"
  Product3/1 -> Matrix Concatenate/2  "DCM10"
  Product4/1 -> Reshape/1  "DCM20"
  Matrix Concatenate/1 -> DCM_normalized/1
  Reshape/1 -> Matrix Concatenate/3

== system AR_Drone_Flight_Control/Navigation/SL3D Visualization/SL3D DCM Output - used to adjust axes to fit wit SL3D convention ==

== system AR_Drone_Flight_Control/Data decomposition to 3D Visualization/SL3D Visualization1/Interchange Axes Mag for SL3D /Home Drone ==
  note: This comes close, however, it doesnt seem that the axis changes properly
      | ie: i rotate drone, the green dot follows it. This  tells me the Z-axis is not
      |  properly placed
  note: y
  note: x
  note: z
  In1 : Inport
  Demux1 : Demux  Outputs=3
  Gain : Gain  Gain=-1
  Gain1 : Gain
  Gain2 : Gain
  Mux2 : Mux  Inputs=3
  Out1 : Outport
  wires:
  Mux2/1 -> Out1/1
  In1/1 -> Demux1/1
  Demux1/3 -> Gain2/1
  Gain2/1 -> Mux2/2
  Demux1/1 -> Gain/1
  Gain/1 -> Mux2/3
  Demux1/2 -> Gain1/1
  Gain1/1 -> Mux2/1

== system AR_Drone_Flight_Control/Data decomposition to 3D Visualization/SL3D Visualization1/Interchange Axes Mag for SL3D /Subsystem ==
  note: This comes close, however, it doesnt seem that the axis changes properly
      | ie: i rotate drone, the green dot follows it. This  tells me the Z-axis is not
      |  properly placed
  note: y
  note: x
  note: z
  In1 : Inport
  Demux1 : Demux  Outputs=3
  Gain : Gain
  Gain1 : Gain  Gain=-1
  Gain2 : Gain  Gain=-1
  Mux2 : Mux  Inputs=3
  Out1 : Outport
  wires:
  Demux1/1 -> Gain2/1
  Gain2/1 -> Mux2/2
  Gain/1 -> Mux2/3
  Gain1/1 -> Mux2/1
  Mux2/1 -> Out1/1
  Demux1/2 -> Gain1/1
  Demux1/3 -> Gain/1
  In1/1 -> Demux1/1

== system AR_Drone_Flight_Control/Data decomposition to 3D Visualization/SL3D Visualization1/Interchange Axes Mag for SL3D /Work Drone ==
  note: This comes close, however, it doesnt seem that the axis changes properly
      | ie: i rotate drone, the green dot follows it. This  tells me the Z-axis is not
      |  properly placed
  note: y
  note: x
  note: z
  In1 : Inport
  Demux1 : Demux  Outputs=3
  Gain : Gain  Gain=-1
  Gain1 : Gain
  Gain2 : Gain
  Mux2 : Mux  Inputs=3
  Out1 : Outport
  wires:
  Mux2/1 -> Out1/1
  In1/1 -> Demux1/1
  Demux1/3 -> Gain2/1
  Gain2/1 -> Mux2/2
  Demux1/1 -> Gain/1
  Gain/1 -> Mux2/3
  Demux1/2 -> Gain1/1
  Gain1/1 -> Mux2/1

== system AR_Drone_Flight_Control/Data decomposition to 3D Visualization/SL3D Visualization1/Interchange Axes Mag for SL3D /Work Drone - supposed work drone .. not really ==
  note: This comes close, however, it doesnt seem that the axis changes properly
      | ie: i rotate drone, the green dot follows it. This  tells me the Z-axis is not
      |  properly placed
  note: y
  note: x
  note: z
  In1 : Inport
  Demux1 : Demux  Outputs=3
  Gain : Gain  Gain=-1
  Gain1 : Gain
  Gain2 : Gain  Gain=-1
  Mux2 : Mux  Inputs=3
  Out1 : Outport
  wires:
  Mux2/1 -> Out1/1
  In1/1 -> Demux1/1
  Demux1/3 -> Gain2/1
  Gain2/1 -> Mux2/2
  Demux1/1 -> Gain/1
  Gain/1 -> Mux2/3
  Demux1/2 -> Gain1/1
  Gain1/1 -> Mux2/1

== system AR_Drone_Flight_Control/Flight Controller/Supervisory Flight Controller/Attitude_Control/Roll Pitch Controller/Low Pass Filter ==
  GyroMeasure : Inport
  Demux : Demux  Outputs=2
  Digital Low Pass Filter1 : DiscreteTransferFcn  Numerator=[0.04877]  Denominator=[1 -0.9512]  OutDataTypeStr=int16
  Digital Low Pass Filter2 : DiscreteTransferFcn  Numerator=[0.04877]  Denominator=[1 -0.9512]  OutDataTypeStr=int16
  Digital Low Pass Filter3 : DiscreteTransferFcn  Commented=on  Numerator=[0.04877]  Denominator=[1 -0.9512]  OutDataTypeStr=int16
  Mux3 : Mux  Inputs=2
  GyroFiltered : Outport
  wires:
  Mux3/1 -> GyroFiltered/1
  Demux/1 -> Digital Low Pass Filter2/1
  GyroMeasure/1 -> Demux/1
  Demux/2 -> Digital Low Pass Filter1/1
  Digital Low Pass Filter2/1 -> Mux3/1
  Digital Low Pass Filter1/1 -> Mux3/2

== system AR_Drone_Flight_Control/Flight Controller/Supervisory Flight Controller/Attitude_Control/Roll Pitch Controller/Outer Loop Euler Angle Control Loop ==
  Attitude_Rate : Inport
  Motor Armed : Inport  Port=2
  Logical Operator : Logic  Operator=NOT  AllPortsSameDT=off  OutDataTypeStr=boolean
  PID Controller : simulink/Continuous/PID Controller  Controller=PID  TimeDomain=Discrete-time  SampleTime=-1  IntegratorMethod=Forward Euler  FilterMethod=Forward Euler  Form=Parallel  P=2.8281  I=28.23  D=0.023379  N=0.0076593  InitialConditionSource=internal  InitialConditionForIntegrator=0  InitialConditionForFilter=0  ExternalReset=level  LimitOutput=on  UpperSaturationLimit=30  LowerSaturationLimit=-30  LinearizeAsGain=on  AntiWindupMode=clamping  Kb=1  TrackingMode=off  Kt=1  PParamMin=[]  PParamMax=[]  IParamMin=[]  IParamMax=[]  DParamMin=[]  DParamMax=[]  NParamMin=[]  NParamMax=[]  KbParamMin=[]  KbParamMax=[]  KtParamMin=[]  KtParamMax=[]  POutMin=[]  POutMax=[]  IOutMin=[]  IOutMax=[]  DOutMin=[]  DOutMax=[]  NOutMin=[]  NOutMax=[]  KbOutMin=[]  KbOutMax=[]  KtOutMin=[]  KtOutMax=[]  IntegratorOutMin=[]  IntegratorOutMax=[]  FilterOutMin=[]  FilterOutMax=[]  SumOutMin=[]  SumOutMax=[]  SumI1OutMin=[]  SumI1OutMax=[]  SumI2OutMin=[]  SumI2OutMax=[]  SumI3OutMin=[]  SumI3OutMax=[]  SumDOutMin=[]  SumDOutMax=[]  SaturationOutMin=[]  SaturationOutMax=[]  IntegratorContinuousStateAttributes=''  IntegratorStateMustResolveToSignalObject=off  IntegratorRTWStateStorageClass=Auto  FilterContinuousStateAttributes=''  FilterStateMustResolveToSignalObject=off  FilterRTWStateStorageClass=Auto
  PID Controller1 : simulink/Continuous/PID Controller  Controller=PID  TimeDomain=Discrete-time  SampleTime=-1  IntegratorMethod=Forward Euler  FilterMethod=Forward Euler  Form=Parallel  P=0.10084*2  I=0.13631*2  D=-0.011755  N=5  InitialConditionSource=internal  InitialConditionForIntegrator=0  InitialConditionForFilter=0  ExternalReset=level  LimitOutput=on  UpperSaturationLimit=30  LowerSaturationLimit=-30  LinearizeAsGain=on  AntiWindupMode=clamping  Kb=1  TrackingMode=off  Kt=1  PParamMin=[]  PParamMax=[]  IParamMin=[]  IParamMax=[]  DParamMin=[]  DParamMax=[]  NParamMin=[]  NParamMax=[]  KbParamMin=[]  KbParamMax=[]  KtParamMin=[]  KtParamMax=[]  POutMin=[]  POutMax=[]  IOutMin=[]  IOutMax=[]  DOutMin=[]  DOutMax=[]  NOutMin=[]  NOutMax=[]  KbOutMin=[]  KbOutMax=[]  KtOutMin=[]  KtOutMax=[]  IntegratorOutMin=[]  IntegratorOutMax=[]  FilterOutMin=[]  FilterOutMax=[]  SumOutMin=[]  SumOutMax=[]  SumI1OutMin=[]  SumI1OutMax=[]  SumI2OutMin=[]  SumI2OutMax=[]  SumI3OutMin=[]  SumI3OutMax=[]  SumDOutMin=[]  SumDOutMax=[]  SaturationOutMin=[]  SaturationOutMax=[]  IntegratorContinuousStateAttributes=''  IntegratorStateMustResolveToSignalObject=off  IntegratorRTWStateStorageClass=Auto  FilterContinuousStateAttributes=''  FilterStateMustResolveToSignalObject=off  FilterRTWStateStorageClass=Auto
  AttitudeRateCmd : Outport
  wires:
  PID Controller1/1 -> AttitudeRateCmd/1  "AttitudeRateCmd"
  Motor Armed/1 -> Logical Operator/1
  Logical Operator/1 -> PID Controller1/2
  Attitude_Rate/1 -> PID Controller1/1

== system AR_Drone_Flight_Control/Navigation/CheckSum Pre-Processing/Accelerometer Processing/Calculate Accel Data ==
  Raw Accel Data : Inport
  Bias : Constant  Value=[0 4096 4096]
  Gain : Gain  Gain=[0.001953125, 0.001953125, 0.001953125]
  Neutral Bias : Constant  Value=[2048 2048 2048]
  Sum : Sum  Inputs=|-+
  Sum1 : Sum  Inputs=|+-
  Processed Accel Data : Outport
  wires:
  Bias/1 -> Sum/2
  Neutral Bias/1 -> Sum1/2
  Sum/1 -> Sum1/1
  Gain/1 -> Processed Accel Data/1
  Sum1/1 -> Gain/1
  Raw Accel Data/1 -> Sum/1

== system AR_Drone_Flight_Control/Navigation/CheckSum Pre-Processing/Accelerometer Processing/CheckSum Correction ==
  CalculatedData : Inport
  CheckSumFlag : Inport  Port=2
  Holding Value : Inport  Port=3
  Compare To Zero : simulink/Logic and Bit Operations/Compare To Zero  relop=>  OutDataTypeStr=boolean
  Delay : Delay  DelayLength=3  InitialCondition=0
  Generate Sample Holding Pulse : Subsystem
  "If True, we have good data, If false, we have bad data, With bad data, use previous good data from N samples ago and hold it on that value for M samples" : Switch  Criteria=u2 > Threshold
  Invert Logic : Logic  Operator=NOT  AllPortsSameDT=off  OutDataTypeStr=boolean
  Logical Operator1 : Logic  Operator=NOT  AllPortsSameDT=off  OutDataTypeStr=boolean
  Pre-Processed Height : Outport
  wires:
  Holding Value/1 -> Generate Sample Holding Pulse/2(HoldDataTicks_Value)
  Invert Logic/1 -> "If True, we have good data, If false, we have bad data, With bad data, use previous good data from N samples ago and hold it on that value for M samples"/2
  Logical Operator1/1 -> Generate Sample Holding Pulse/1(CheckSumFlag)
  Generate Sample Holding Pulse/1(Hold_Data_Pulse) -> Invert Logic/1
  Compare To Zero/1 -> Logical Operator1/1
  Delay/1 -> "If True, we have good data, If false, we have bad data, With bad data, use previous good data from N samples ago and hold it on that value for M samples"/3
  "If True, we have good data, If false, we have bad data, With bad data, use previous good data from N samples ago and hold it on that value for M samples"/1 -> Delay/1, Pre-Processed Height/1
  CalculatedData/1 -> "If True, we have good data, If false, we have bad data, With bad data, use previous good data from N samples ago and hold it on that value for M samples"/1
  CheckSumFlag/1 -> Compare To Zero/1

== system AR_Drone_Flight_Control/Navigation/CheckSum Pre-Processing/Magnetometer/CheckSum Correction ==
  CalculatedData : Inport
  CheckSumFlag : Inport  Port=2
  Holding Value : Inport  Port=3
  Compare To Zero : simulink/Logic and Bit Operations/Compare To Zero  relop=>  OutDataTypeStr=boolean
  Delay : Delay  DelayLength=3  InitialCondition=0
  Generate Sample Holding Pulse : Subsystem
  "If True, we have good data, If false, we have bad data, With bad data, use previous good data from N samples ago and hold it on that value for M samples" : Switch  Criteria=u2 > Threshold
  Invert Logic : Logic  Operator=NOT  AllPortsSameDT=off  OutDataTypeStr=boolean
  Logical Operator1 : Logic  Operator=NOT  AllPortsSameDT=off  OutDataTypeStr=boolean
  Pre-Processed Data : Outport
  wires:
  Holding Value/1 -> Generate Sample Holding Pulse/2(HoldDataTicks_Value)
  Invert Logic/1 -> "If True, we have good data, If false, we have bad data, With bad data, use previous good data from N samples ago and hold it on that value for M samples"/2
  Logical Operator1/1 -> Generate Sample Holding Pulse/1(CheckSumFlag)
  Generate Sample Holding Pulse/1(Hold_Data_Pulse) -> Invert Logic/1
  Compare To Zero/1 -> Logical Operator1/1
  Delay/1 -> "If True, we have good data, If false, we have bad data, With bad data, use previous good data from N samples ago and hold it on that value for M samples"/3
  "If True, we have good data, If false, we have bad data, With bad data, use previous good data from N samples ago and hold it on that value for M samples"/1 -> Delay/1, Pre-Processed Data/1
  CalculatedData/1 -> "If True, we have good data, If false, we have bad data, With bad data, use previous good data from N samples ago and hold it on that value for M samples"/1
  CheckSumFlag/1 -> Compare To Zero/1

== system AR_Drone_Flight_Control/Navigation/CheckSum Pre-Processing/Magnetometer/Process Raw Mag Data ==
  note: magnetometer[ 0 ] = - ( float ) navdata.mx ;
      | magnetometer[ 1 ] = ( float ) navdata.my ;
      | magnetometer[ 2 ] = - ( float ) navdata.mz ;
      | const float Sensitivity[ 3 ] = { 0.0071492608 , 0.0070882491 , 0.0074057781 } ;
      | const float Neutral[ 3 ] = { 118.0 , - 65.0 , 110.0 } ;
  Magnetometer : Inport
  Bias : Constant  Value=[ 118.0, -65.0, 110.0 ]
  Sum : Sum  Inputs=|+-
  postGain : Gain  Gain=[0.0071492608, 0.0070882491, 0.0074057781]
  preGain : Gain  Gain=[-1 1 -1]
  ProcessedData : Outport
  wires:
  Bias/1 -> Sum/2
  preGain/1 -> Sum/1
  Sum/1 -> postGain/1
  Magnetometer/1 -> preGain/1
  postGain/1 -> ProcessedData/1

== system AR_Drone_Flight_Control/Navigation/CheckSum Pre-Processing/RateGyro Processing/CheckSum Correction ==
  CalculatedData : Inport
  CheckSumFlag : Inport  Port=2
  Holding Value : Inport  Port=3
  Compare To Zero : simulink/Logic and Bit Operations/Compare To Zero  relop=>  OutDataTypeStr=boolean
  Delay : Delay  DelayLength=3  InitialCondition=0
  Generate Sample Holding Pulse : Subsystem
  "If True, we have good data, If false, we have bad data, With bad data, use previous good data from N samples ago and hold it on that value for M samples" : Switch  Criteria=u2 > Threshold
  Invert Logic : Logic  Operator=NOT  AllPortsSameDT=off  OutDataTypeStr=boolean
  Logical Operator1 : Logic  Operator=NOT  AllPortsSameDT=off  OutDataTypeStr=boolean
  Pre-Processed Height : Outport
  wires:
  Holding Value/1 -> Generate Sample Holding Pulse/2(HoldDataTicks_Value)
  Invert Logic/1 -> "If True, we have good data, If false, we have bad data, With bad data, use previous good data from N samples ago and hold it on that value for M samples"/2
  Logical Operator1/1 -> Generate Sample Holding Pulse/1(CheckSumFlag)
  Generate Sample Holding Pulse/1(Hold_Data_Pulse) -> Invert Logic/1
  Compare To Zero/1 -> Logical Operator1/1
  Delay/1 -> "If True, we have good data, If false, we have bad data, With bad data, use previous good data from N samples ago and hold it on that value for M samples"/3
  "If True, we have good data, If false, we have bad data, With bad data, use previous good data from N samples ago and hold it on that value for M samples"/1 -> Delay/1, Pre-Processed Height/1
  CalculatedData/1 -> "If True, we have good data, If false, we have bad data, With bad data, use previous good data from N samples ago and hold it on that value for M samples"/1
  CheckSumFlag/1 -> Compare To Zero/1

== system AR_Drone_Flight_Control/Navigation/CheckSum Pre-Processing/RateGyro Processing/Process Data ==
  note: const float Sensitivity[ 3 ] = { 0.0609 , 0.0609 , 0.0609 } ;
      | const float Neutral[ 3 ] = { 0.0 , 0.0 , 0.0 } ;
      | const int16_t Offset[ 3 ] = { - 73 , 14 , - 13 } ;
      | const int16_t Noises[ 3 ] = { 35 , 35 , 15 } ;
      |
      | int16_t vRaws[ 3 ] = {
      | Navdata :: IMU :: Gyroscope :: getRawX (),
      | Navdata :: IMU :: Gyroscope :: getRawY (),
      | Navdata :: IMU :: Gyroscope :: getRawZ ()
      | } ;
      |
      | gyroscope[i] = vRaws[i] * Gyroscope :: Sensitivity[i] * M_PI / 180.0 ;
  Raw Data : Inport
  Constant : Constant  Value=[0.0, 0.0, 0.0]
  Gain : Gain  Gain=[0.0609, 0.0609, 0.0609]
  Sum : Sum  Inputs=|++
  Processed Data : Outport
  wires:
  Raw Data/1 -> Sum/1
  Constant/1 -> Sum/2
  Gain/1 -> Processed Data/1
  Sum/1 -> Gain/1

== system AR_Drone_Flight_Control/Navigation/CheckSum Pre-Processing/TempFilter/CheckSum Correction ==
  CalculatedData : Inport
  CheckSumFlag : Inport  Port=2
  Holding Value : Inport  Port=3
  Compare To Zero : simulink/Logic and Bit Operations/Compare To Zero  relop=>  OutDataTypeStr=boolean
  Delay : Delay  DelayLength=3  InitialCondition=0
  Generate Sample Holding Pulse : Subsystem
  "If True, we have good data, If false, we have bad data, With bad data, use previous good data from N samples ago and hold it on that value for M samples" : Switch  Criteria=u2 > Threshold
  Invert Logic : Logic  Operator=NOT  AllPortsSameDT=off  OutDataTypeStr=boolean
  Logical Operator1 : Logic  Operator=NOT  AllPortsSameDT=off  OutDataTypeStr=boolean
  Pre-Processed Data : Outport
  wires:
  Holding Value/1 -> Generate Sample Holding Pulse/2(HoldDataTicks_Value)
  Invert Logic/1 -> "If True, we have good data, If false, we have bad data, With bad data, use previous good data from N samples ago and hold it on that value for M samples"/2
  Logical Operator1/1 -> Generate Sample Holding Pulse/1(CheckSumFlag)
  Generate Sample Holding Pulse/1(Hold_Data_Pulse) -> Invert Logic/1
  Compare To Zero/1 -> Logical Operator1/1
  Delay/1 -> "If True, we have good data, If false, we have bad data, With bad data, use previous good data from N samples ago and hold it on that value for M samples"/3
  "If True, we have good data, If false, we have bad data, With bad data, use previous good data from N samples ago and hold it on that value for M samples"/1 -> Delay/1, Pre-Processed Data/1
  CalculatedData/1 -> "If True, we have good data, If false, we have bad data, With bad data, use previous good data from N samples ago and hold it on that value for M samples"/1
  CheckSumFlag/1 -> Compare To Zero/1

== system AR_Drone_Flight_Control/Navigation/CheckSum Pre-Processing/TempFilter/Process Raw Mag Data ==
  note: magnetometer[ 0 ] = - ( float ) navdata.mx ;
      | magnetometer[ 1 ] = ( float ) navdata.my ;
      | magnetometer[ 2 ] = - ( float ) navdata.mz ;
      | const float Sensitivity[ 3 ] = { 0.0071492608 , 0.0070882491 , 0.0074057781 } ;
      | const float Neutral[ 3 ] = { 118.0 , - 65.0 , 110.0 } ;
  Magnetometer : Inport
  Bias : Constant  Value=[ 118.0, -65.0, 110.0 ]
  Sum : Sum  Inputs=|+-
  postGain : Gain  Gain=[0.0071492608, 0.0070882491, 0.0074057781]
  preGain : Gain  Gain=[-1 1 -1]
  ProcessedData : Outport
  wires:
  Bias/1 -> Sum/2
  preGain/1 -> Sum/1
  Sum/1 -> postGain/1
  Magnetometer/1 -> preGain/1
  postGain/1 -> ProcessedData/1

== system AR_Drone_Flight_Control/Navigation/CheckSum Pre-Processing/Ultrasound Processing/CheckSum Correction ==
  CalculatedData : Inport
  CheckSumFlag : Inport  Port=2
  Holding Value : Inport  Port=3
  Compare To Zero : simulink/Logic and Bit Operations/Compare To Zero  relop=>  OutDataTypeStr=boolean
  Delay : Delay  DelayLength=3  InitialCondition=0
  Generate Sample Holding Pulse : Subsystem
  "If True, we have good data, If false, we have bad data, With bad data, use previous good data from N samples ago and hold it on that value for M samples" : Switch  Criteria=u2 > Threshold
  Invert Logic : Logic  Operator=NOT  AllPortsSameDT=off  OutDataTypeStr=boolean
  Logical Operator1 : Logic  Operator=NOT  AllPortsSameDT=off  OutDataTypeStr=boolean
  Pre-Processed Height : Outport
  wires:
  Holding Value/1 -> Generate Sample Holding Pulse/2(HoldDataTicks_Value)
  Invert Logic/1 -> "If True, we have good data, If false, we have bad data, With bad data, use previous good data from N samples ago and hold it on that value for M samples"/2
  Logical Operator1/1 -> Generate Sample Holding Pulse/1(CheckSumFlag)
  Generate Sample Holding Pulse/1(Hold_Data_Pulse) -> Invert Logic/1
  Compare To Zero/1 -> Logical Operator1/1
  Delay/1 -> "If True, we have good data, If false, we have bad data, With bad data, use previous good data from N samples ago and hold it on that value for M samples"/3
  "If True, we have good data, If false, we have bad data, With bad data, use previous good data from N samples ago and hold it on that value for M samples"/1 -> Delay/1, Pre-Processed Height/1
  CalculatedData/1 -> "If True, we have good data, If false, we have bad data, With bad data, use previous good data from N samples ago and hold it on that value for M samples"/1
  CheckSumFlag/1 -> Compare To Zero/1

== system AR_Drone_Flight_Control/Navigation/Data Conversion and Measurement Calculation/Calculate Gravity Vector/Accelerometer Neutral Gain and Offset ==
  note: (1/512)g /LSB
  note: All axes were invereted here, both implementations in paparazzi and student team seem to do this
  Raw Accel Data : Inport
  Bias : Constant  Value=[4096]
  Data Type Conversion : DataTypeConversion  OutDataTypeStr=int16
  Demux : Demux  Outputs=3
  Gain : Gain  Gain=1/512
  Gain1 : Gain  Gain=-1  OutDataTypeStr=double
  Gain2 : Gain  Gain=-1  OutDataTypeStr=double
  Gain3 : Gain  Gain=-1  OutDataTypeStr=double
  Mux : Mux  Inputs=3
  Neutral Bias : Constant  Value=[2048 2048 2048]
  Sum : Sum  Inputs=|++
  Sum1 : Sum  Inputs=|+-
  Sum2 : Sum  Inputs=|++
  Sum3 : Sum  Inputs=|++
  Processed Accel Data : Outport
  wires:
  Gain1/1 -> Sum3/1
  Data Type Conversion/1 -> Demux/1
  Bias/1 -> Sum3/2, Sum/2, Sum2/2
  Sum2/1 -> Mux/3
  Gain3/1 -> Sum2/1
  Demux/3 -> Gain3/1
  Sum/1 -> Mux/2
  Gain2/1 -> Sum/1
  Demux/2 -> Gain2/1
  Sum3/1 -> Mux/1
  Demux/1 -> Gain1/1
  Raw Accel Data/1 -> Data Type Conversion/1
  Neutral Bias/1 -> Sum1/2
  Mux/1 -> Sum1/1
  Gain/1 -> Processed Accel Data/1
  Sum1/1 -> Gain/1
